simulink model "Driver_CS9"  (R2018b)
settings: Solver=ode45  StartTime=0  StopTime=100  FixedStep=0.002  RelTol=1e-3  AbsTol=1e-6
PreLoadFcn:
  | routing_planning;
  | K_calculation;
undefined symbols (not defined in the file): a, b, Cf, Cr, Iz, kappar, m, thetar, xr, yr
libraries: Solver_SF x1
settings Model: ExtModeTrigMode=oneshot  ExtModeArmWhenConnect=off  Creator=dhall  LastModifiedBy=wxmjy
settings SolverCC: AutoScaleAbsTol=off
settings DataIOCC: SaveFormat=Array  SignalLoggingSaveFormat=ModelDataLogs  SignalLoggingName=sigsOut
settings OptimizationCC: BooleanDataType=off  ExpressionDepthLimit=2147483647  InitFltsAndDblsToZero=on  LifeSpan=inf
settings DebuggingCC: SaveWithParameterizedLinksMsg=none  UnderspecifiedInitializationDetection=Classic  MergeDetectMultiDrivingBlocksExec=none  SignalResolutionControl=TryResolveAllWithWarning  MultiTaskDSMMsg=warning  MultiTaskCondExecSysMsg=none  FcnCallInpInsideContextMsg=warning  StateNameClashWarn=warning  SFUnexpectedBacktrackingDiag=warning  SFNoUnconditionalDefaultTransitionDiag=warning  SFExecutionAtInitializationDiag=none
settings HardwareCC: ProdBitPerPointer=32  ProdBitPerSizeT=32  ProdBitPerPtrDiffT=32  ProdLargestAtomicFloat=None  ProdIntDivRoundTo=Undefined  ProdEndianess=Unspecified  ProdWordSize=32  ProdHWDeviceType=32-bit Generic  TargetUnknown=on
settings ModelReferenceCC: PropagateSignalLabelsOutOfModel=off
settings SFSimCC: SimUseLocalCustomCode=off
settings RTWCC: TemplateMakefile=grt_vc.tmf  RTWUseLocalCustomCode=off
settings CodeAppCC: StateflowObjectComments=on
settings GRTTargetCC: TargetFcnLib=ansi_tfl_tmw.mat  TargetLangStandard=C89/C90 (ANSI)  ModelReferenceCompliant=off  GeneratePreprocessorConditionals=Disable all  CombineOutputUpdateFcns=off  MatFileLogging=off  GRTInterface=on
settings ConfigComp: CovMetricSettings=dw  CovHtmlReporting=on  CovSaveCumulativeToWorkspaceVar=on  CovSaveSingleToWorkspaceVar=on  CovExternalEMLEnable=off

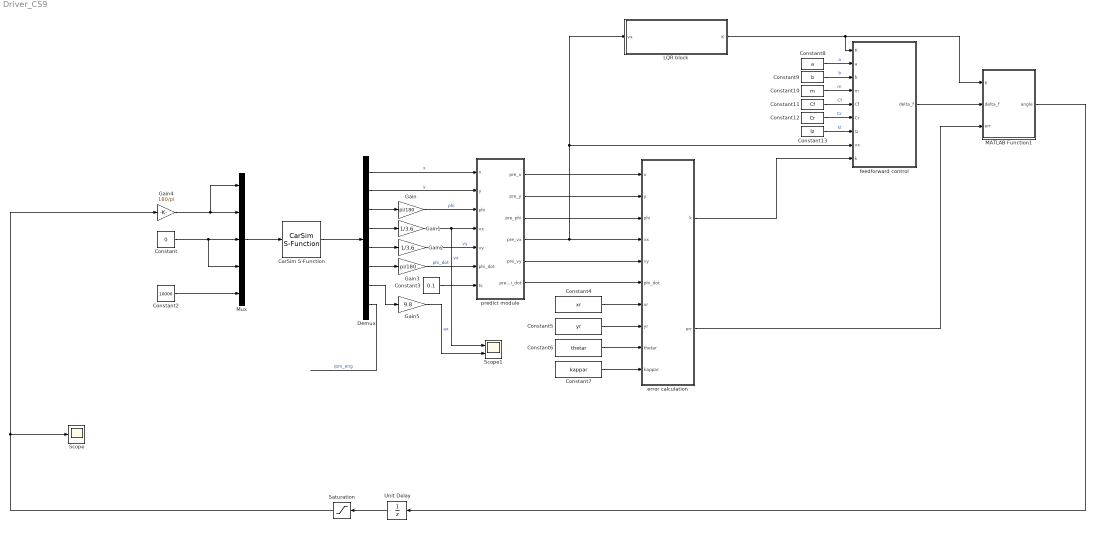
== system Driver_CS9 ==
  CarSim S-Function : Solver_SF/CarSim S-Function  Priority=1  SIMFILE=simfile.sim  Run_RTs=off  vs_state_ind=Run  StopMode_ind=Vehicle Model
  Constant : Constant  Value=0
  Constant10 : Constant  Value=m
  Constant11 : Constant  Value=Cf
  Constant12 : Constant  Value=Cr
  Constant13 : Constant  Value=Iz
  Constant2 : Constant  Value=10000
  Constant3 : Constant  Value=0.1
  Constant4 : Constant  Value=xr
  Constant5 : Constant  Value=yr
  Constant6 : Constant  Value=thetar
  Constant7 : Constant  Value=kappar
  Constant8 : Constant  Value=a
  Constant9 : Constant  Value=b
  Demux : Demux  Outputs=8
  Gain : Gain  Gain=pi/180
  Gain1 : Gain  Gain=1/3.6
  Gain2 : Gain  Gain=1/3.6
  Gain3 : Gain  Gain=pi/180
  Gain4 : Gain  Gain=180/pi
  Gain5 : Gain  Gain=9.8
  LQR block : Subsystem
  MATLAB Function1 : MATLAB Function  TreatAsAtomicUnit=on
  Mux : Mux  Inputs=5
  Saturation : Saturate  UpperLimit=1.2  LowerLimit=-1.2
  Scope : Scope
  Scope1 : Scope  NumInputPorts=2
  Unit Delay : UnitDelay  SampleTime=-1
  error calculation : MATLAB Function  TreatAsAtomicUnit=on
  feedforward control : MATLAB Function  TreatAsAtomicUnit=on
  predict module : MATLAB Function  TreatAsAtomicUnit=on
  wires:
  Mux/1 -> CarSim S-Function/1
  CarSim S-Function/1 -> Demux/1
  Constant2/1 -> Mux/5
  Constant/1 -> Mux/3, Mux/4
  MATLAB Function1/1(angle) -> Unit Delay/1
  Demux/1 -> predict module/1(x)  "x"
  Demux/2 -> predict module/2(y)  "y"
  Demux/3 -> Gain/1
  Demux/4 -> Gain1/1
  Demux/5 -> Gain2/1
  Demux/6 -> Gain3/1
  Gain/1 -> predict module/3(phi)  "phi"
  Gain1/1 -> Scope1/1, predict module/4(vx)  "vx"
  Gain2/1 -> predict module/5(vy)  "vy"
  Gain3/1 -> predict module/6(phi_dot)  "phi_dot"
  Constant3/1 -> predict module/7(ts)
  predict module/1(pre_x) -> error calculation/1(x)
  predict module/2(pre_y) -> error calculation/2(y)
  predict module/3(pre_phi) -> error calculation/3(phi)
  predict module/4(pre_vx) -> error calculation/4(vx), LQR block/1(vx), feedforward control/8(vx)
  predict module/5(pre_vy) -> error calculation/5(vy)
  predict module/6(pre_phi_dot) -> error calculation/6(phi_dot)
  Constant4/1 -> error calculation/7(xr)
  Constant7/1 -> error calculation/10(kappar)
  Constant6/1 -> error calculation/9(thetar)
  Constant5/1 -> error calculation/8(yr)
  error calculation/1(k) -> feedforward control/9(k)
  Constant8/1 -> feedforward control/2(a)  "a"
  Constant13/1 -> feedforward control/7(Iz)  "Iz"
  Constant12/1 -> feedforward control/6(Cr)  "Cr"
  Constant11/1 -> feedforward control/5(Cf)  "Cf"
  Constant10/1 -> feedforward control/4(m)  "m"
  Constant9/1 -> feedforward control/3(b)  "b"
  LQR block/1(K) -> MATLAB Function1/1(K), feedforward control/1(K)
  feedforward control/1(delta_f) -> MATLAB Function1/2(delta_f)
  error calculation/2(err) -> MATLAB Function1/3(err)
  Gain4/1 -> Mux/2, Mux/1
  Unit Delay/1 -> Saturation/1
  Saturation/1 -> Scope/1, Gain4/1
  Demux/7 -> Gain5/1
  Demux/8 -> ?  "rpm_eng"
  Gain5/1 -> Scope1/2  "ax"

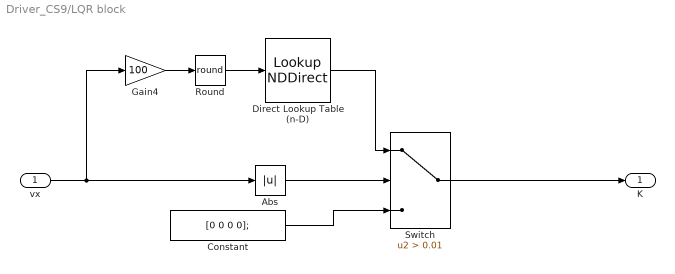
== system Driver_CS9/LQR block ==
  vx : Inport
  Abs : Abs
  Constant : Constant  Value=[0 0 0 0];  VectorParams1D=off
  Direct Lookup Table (n-D) : LookupNDDirect  InputsSelectThisObjectFromTable=Vector  Table=K'
  Gain4 : Gain  Gain=100
  Round : Rounding  Operator=round
  Switch : Switch  Criteria=u2 > Threshold  Threshold=0.01
  K : Outport
  wires:
  Direct Lookup Table (n-D)/1 -> Switch/1
  Gain4/1 -> Round/1
  Round/1 -> Direct Lookup Table (n-D)/1
  vx/1 -> Gain4/1, Abs/1
  Abs/1 -> Switch/2
  Constant/1 -> Switch/3
  Switch/1 -> K/1

== matlab function Driver_CS9/error calculation ==
  data: x input; k output; y input; phi input; vx input; vy input; phi_dot input; xr input; yr input; thetar input; kappar input; err output
function [k, err] = fcn(x, y, phi, vx, vy, phi_dot, xr, yr, thetar, kappar)

% find the closest planning point
[val, ind] = min((x-xr).^2 + (y-yr).^2);

% calcualte the tangent and normal vectors
tau = [cos(thetar(ind)), sin(thetar(ind))];
n   = [-sin(thetar(ind)), cos(thetar(ind))];

d_e = [x-xr(ind), y-yr(ind)];

ed = n * d_e';

es = tau * d_e';

% pro_point_thetar = thetar(ind); % apollo
pro_point_thetar = thetar(ind) + kappar(ind)*es; 

ed_dot = vy * cos(phi-pro_point_thetar) + vx * sin(phi-pro_point_thetar);

e_phi = sin(phi - pro_point_thetar); % sin为了消除多值性

s_dot = (vx*cos(phi-pro_point_thetar) - vy*sin(phi-pro_point_thetar)) / (1-kappar(ind)*ed);

e_phi_dot = phi_dot - kappar(ind)*s_dot;

k = kappar(ind);
err = [ed, ed_dot, e_phi, e_phi_dot];

end

== matlab function Driver_CS9/predict module ==
  data: x input; pre_x output; y input; phi input; vx input; vy input; phi_dot input; ts input; pre_y output; pre_phi output; pre_vx output; pre_vy output; pre_phi_dot output
function [pre_x, pre_y, pre_phi, pre_vx, pre_vy, pre_phi_dot] = fcn(x, y, phi, vx, vy, phi_dot, ts)
pre_x       = x + vx*ts*cos(phi) - vy*ts*sin(phi);
pre_y       = y + vy*ts*cos(phi) + vx*ts*sin(phi);
pre_phi     = phi + phi_dot*ts;
pre_vx      = vx;
pre_vy      = vy;
pre_phi_dot = phi_dot;
end

== matlab function Driver_CS9/feedforward control ==
  data: K input; delta_f output; a input; b input; m input; Cf input; Cr input; Iz input; vx input; k input
function delta_f = fcn(K, a,b,m,Cf,Cr,Iz, vx, k)
K3 = K(3);

delta_f = k * (a + b - b*K3 ...
    - (m*vx^2)/(a+b)*(b/Cf + a/Cr*K3 - a/Cr));
end

== matlab function Driver_CS9/MATLAB Function1 ==
  data: K input; angle output; delta_f input; err input
function angle = fcn(K, delta_f, err)

angle = -K*err'+delta_f;
